simulink model "lab2sim"  (R2023a)
settings: Solver=VariableStepAuto  StartTime=0.0  StopTime=20  RelTol=1e-3
settings Model: Creator=yer2  LastModifiedBy=yer2

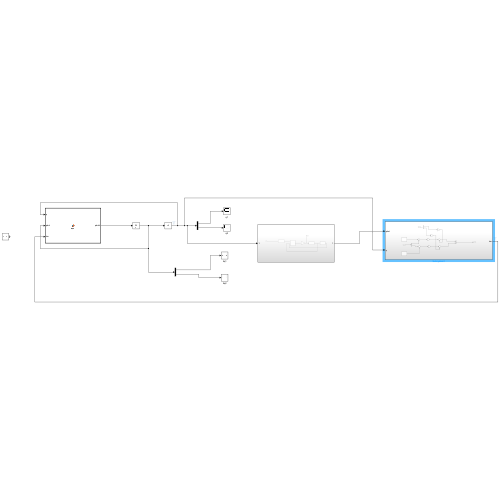
[thumbnail: Simulink's stored preview of the top-level diagram]
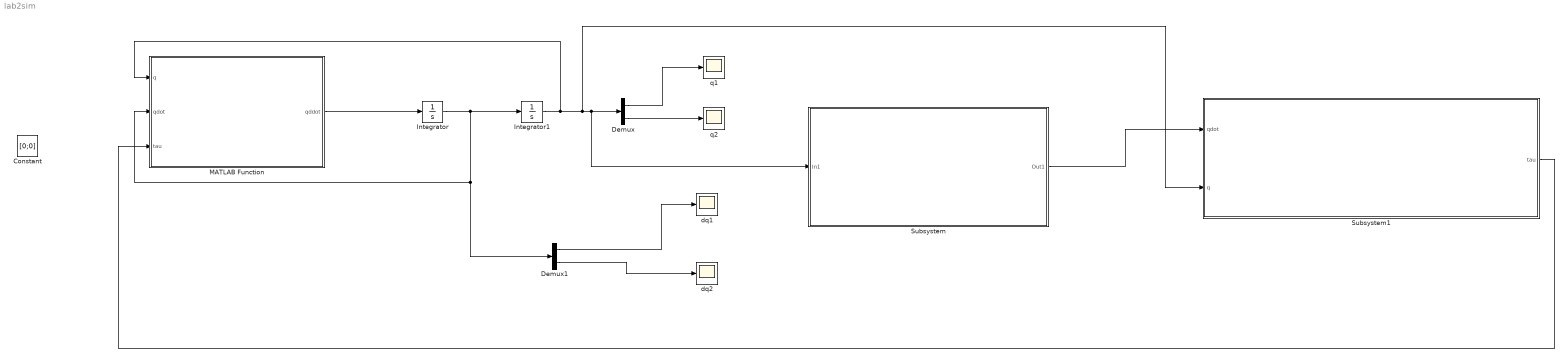
== system lab2sim ==
  Constant : Constant  Value=[0;0]
  Demux : Demux  Outputs=2
  Demux1 : Demux  Outputs=2
  Integrator : Integrator  InitialCondition=[0;0]
  Integrator1 : Integrator  InitialCondition=[0;0]
  MATLAB Function : MATLAB Function  TreatAsAtomicUnit=on
  Subsystem : Subsystem
  Subsystem1 : Subsystem
  dq1 : Scope
  dq2 : Scope
  q1 : Scope
  q2 : Scope
  wires:
  MATLAB Function/1(qddot) -> Integrator/1
  Demux/2 -> q2/1
  Demux/1 -> q1/1
  Demux1/1 -> dq1/1
  Demux1/2 -> dq2/1
  Integrator/1 -> Demux1/1, MATLAB Function/2(qdot), Integrator1/1
  Subsystem/1(Out1) -> Subsystem1/1(qdot)
  Integrator1/1 -> MATLAB Function/1(q), Subsystem1/2(q), Subsystem/1(In1), Demux/1
  Subsystem1/1(tau) -> MATLAB Function/3(tau)

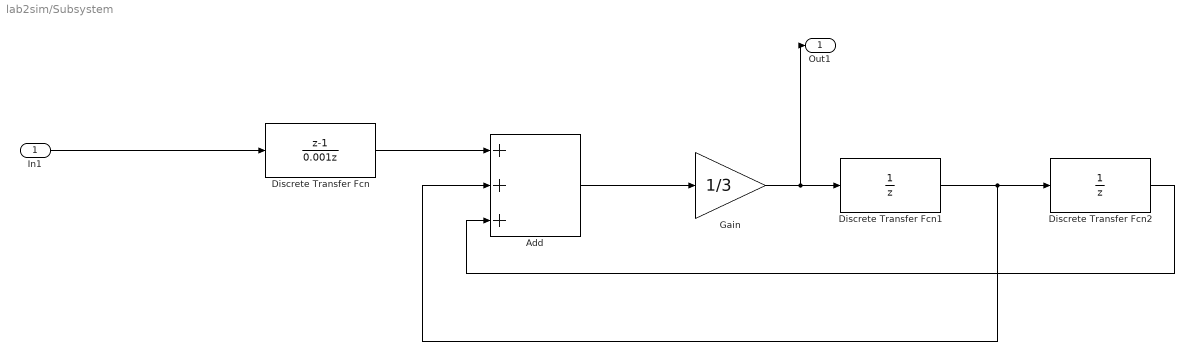
== system lab2sim/Subsystem ==
  In1 : Inport
  Add : Sum  Inputs=+++
  Discrete Transfer Fcn : DiscreteTransferFcn  Numerator=[1 -1]  Denominator=[0.001 0]
  Discrete Transfer Fcn1 : DiscreteTransferFcn  Denominator=[1 0]
  Discrete Transfer Fcn2 : DiscreteTransferFcn  Denominator=[1 0]
  Gain : Gain  Gain=1/3
  Out1 : Outport
  wires:
  Add/1 -> Gain/1
  Discrete Transfer Fcn/1 -> Add/1
  Discrete Transfer Fcn2/1 -> Add/3
  Discrete Transfer Fcn1/1 -> Add/2, Discrete Transfer Fcn2/1
  Gain/1 -> Out1/1, Discrete Transfer Fcn1/1
  In1/1 -> Discrete Transfer Fcn/1

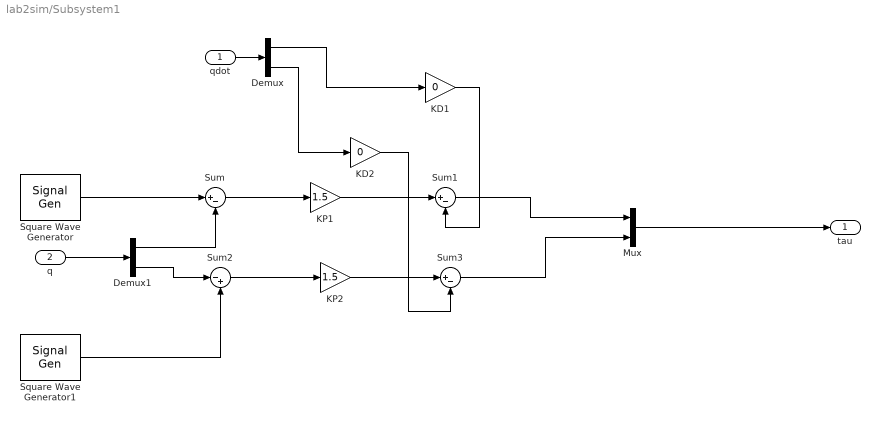
== system lab2sim/Subsystem1 ==
  qdot : Inport
  q : Inport  Port=2
  Demux : Demux  Outputs=2
  Demux1 : Demux  Outputs=2
  KD1 : Gain  Gain=0
  KD2 : Gain  Gain=0
  KP1 : Gain  Gain=1.5
  KP2 : Gain  Gain=1.5
  Mux : Mux  Inputs=2
  Square Wave Generator : SignalGenerator  WaveForm=square  Amplitude=pi/6
  Square Wave Generator1 : SignalGenerator  WaveForm=square  Amplitude=pi/6
  Sum : Sum  Inputs=|+-
  Sum1 : Sum  Inputs=|+-
  Sum2 : Sum  Inputs=|-+
  Sum3 : Sum  Inputs=|+-
  tau : Outport
  wires:
  qdot/1 -> Demux/1
  q/1 -> Demux1/1
  Square Wave Generator/1 -> Sum/1
  Demux1/1 -> Sum/2
  Sum/1 -> KP1/1
  KP1/1 -> Sum1/1
  Sum1/1 -> Mux/1
  Mux/1 -> tau/1
  Demux1/2 -> Sum2/1
  Square Wave Generator1/1 -> Sum2/2
  Sum2/1 -> KP2/1
  KP2/1 -> Sum3/1
  Sum3/1 -> Mux/2
  Demux/1 -> KD1/1
  KD1/1 -> Sum1/2
  Demux/2 -> KD2/1
  KD2/1 -> Sum3/2

== matlab function lab2sim/MATLAB Function ==
  data: q input; qdot input; tau input; qddot output
function qddot = fcn(q, qdot, tau)

theta2M = q(1);
theta3M = q(2);
theta2M_dot = qdot(1);
theta3M_dot = qdot(2);
g = 9.81;
p = [0.0300;0.0128;0.0076;0.0753;0.0298];
D_theta = [p(1), -p(3)*sin(theta3M - theta2M);
           -p(3)*sin(theta3M - theta2M), p(2)];

C_theta = [0, -p(3)*cos(theta3M - theta2M)*theta3M_dot;
           p(3)*cos(theta3M - theta2M)*theta2M_dot, 0];
G_theta = [-p(4)*g*sin(theta2M);
           -p(5)*g*cos(theta3M)];

qddot = D_theta\(tau-C_theta*qdot-G_theta);
